simulink model "guidance"  (R2021b)
settings: Solver=VariableStepAuto  StartTime=0.0  StopTime=50  RelTol=1e-3
values from neighbouring files (symbols this model uses):
  A_R = b^2/S    (= 3.125)    [tailsitterParam.m]
  b = [b1;b2;b3;b4;b5;b4;b3]    [tailsitterParam.m]
  c = [c1;c2;c3;c3;c3;c3;c3]    [tailsitterParam.m]
  C_D0 = 0.02    [tailsitterParam.m]
  C_D_R = 1.1    [tailsitterParam.m]
  C_M_coeff = polyfit(C_M_alpha(:,1), C_M_alpha(:,2),3)    [tailsitterParam.m]
  Cl_alpha = (2*pi*cos(Lambda))/(2*cos(Lambda)/A_R + sqrt(1 + (2*cos(Lambda)/A_R)^2))    [tailsitterParam.m]
  d = cat(2,p_d,p_d)    [tailsitterParam.m]
  g = -9.82    [tailsitterParam.m]
  Ic = [Ix 0 -Ixz;0 Iy 0;-Ixz 0 Iz]    [tailsitterParam.m]
  INIT_ETA = [0.5;0;0.5;axang2quat([0 1 0 -1.572])']    [guidanceParams.m]
  Ith = 1.6*10^(-6)    (= 1.6e-06)    [tailsitterParam.m]
  k0 = 0.87    [tailsitterParam.m]
  Kp_o = eye(3)*2    [controllerParams.m]
  Kp_p = eye(3)*5    [controllerParams.m]
  Kv_o = eye(3)*3    [controllerParams.m]
  Kv_p = eye(3)*3    [controllerParams.m]
  l = 0.145    [tailsitterParam.m]
  li = cat(2,lr,ll)    [tailsitterParam.m]
  m = 0.21    [tailsitterParam.m]
  M = [m * eye(3,3) zeros(3,3);zeros(3,3) Ic]    [tailsitterParam.m]
  M_inv = inv(M)    [tailsitterParam.m]
  Omega_max = 1500    [tailsitterParam.m]
  pm = cat(2,prm,plm)    [tailsitterParam.m]
  r_B = r_B./1000    [tailsitterParam.m]
  R_eleb1 = axang2rotm([0 0 1 -0.16349])    [tailsitterParam.m]
  R_eleb2 = axang2rotm([0 0 1 0.15331])    [tailsitterParam.m]
  rho = 1.225    [tailsitterParam.m]
  rp = 0.0625    [tailsitterParam.m]
  rv_B = rv_B./1000    [tailsitterParam.m]
  SLERP_a = flip(SLERP_B \ SLERP_bconstraints)    [guidanceParams.m]
  tf_a = [(1/wn) (1+2*damp) (1+2*damp)*wn wn^2]    [guidanceParams.m]
  tf_b = [wn^2]    [guidanceParams.m]
  wpts = [wpts_p;wpts_qs]    [guidanceParams.m]
libraries: simulink_extras x3, simulink x2, dspswit3 x1, vrlib x1
settings Model: Creator=Thobi  LastModifiedBy=Thobi

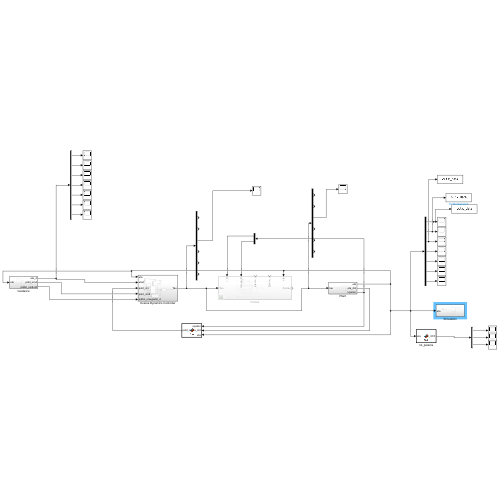
[thumbnail: Simulink's stored preview of the top-level diagram]
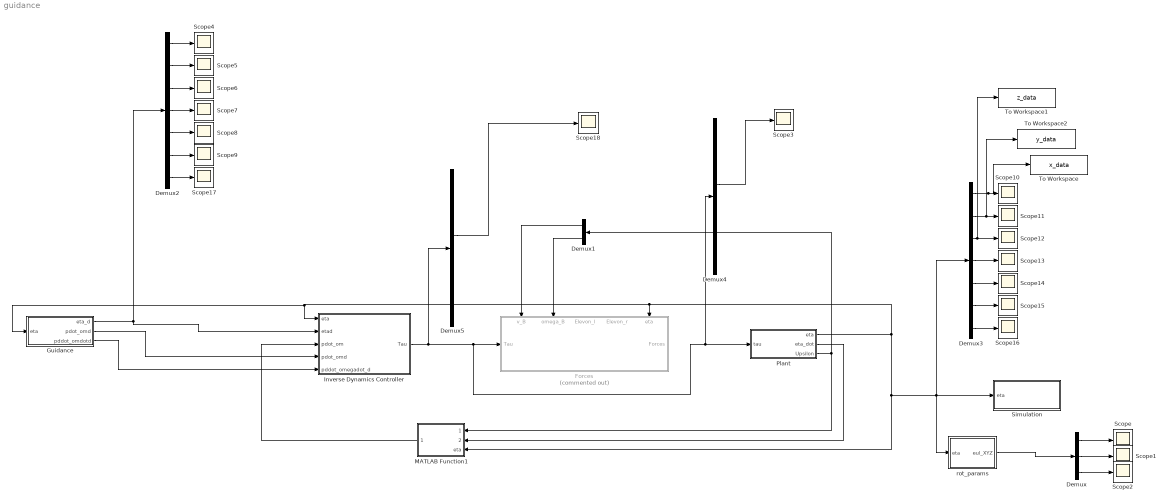
== system guidance ==
  Demux : Demux  Outputs=3
  Demux1 : Demux  Outputs=2
  Demux2 : Demux  Outputs=7
  Demux3 : Demux  Outputs=7
  Demux4 : Demux  Outputs=6
  Demux5 : Demux  Outputs=6
  Forces : Subsystem  Commented=on
      settings: PortSchema="{\"entries\":[{\"content\":{\"sides\":[{\"content\":{\"connectorIds\":[\"In1\"]},\"type\":\"ConnectorPlacement.EquallySpacedRectSide\",\"uuid\":\"b69eaf1b-34d3-48b5-a479-e73058574737\"},{\"content\":{\"connectorIds\":[\"Out1\"],\"side\":\"RIGHT\"},\"type\":\"ConnectorPlacement.EquallySpacedRectSide\",\"uuid\":\"360c4a31-c3bb-45fe-b4f9-363a1910a025\"},{\"content\":{\"connectorIds\":[\"In2\",\"In3\",\"In4\",\"In5\",\"In6\"],\"side\":\"TOP\"},\"type\":\"ConnectorPlacement.EquallySpacedRectSide\",\"uuid\":\"c1210f58-2836-4525-bf47-18b3ef4457c4\"}]},\"type\":\"ConnectorPlacement.EquallySpacedConnector\",\"uuid\":\"84dfde55-8f7b-46f6-8c53-c0c170e7b308\"}],\"packageUris\":[\"http://schema.mathworks.com/mf0/Connector/R2020b\"],\"version\":\"1.0\"}"
  Guidance : Subsystem
  Inverse Dynamics Controller : Subsystem
  MATLAB Function1 : MATLAB Function  TreatAsAtomicUnit=on
  Plant : Subsystem
  Scope{,1..18} (19 alike) : Scope
  Simulation : Subsystem
  To Workspace : ToWorkspace  VariableName=x_data  SaveFormat=Timeseries  SampleTime=-1
  To Workspace1 : ToWorkspace  VariableName=z_data  SaveFormat=Timeseries  SampleTime=-1
  To Workspace2 : ToWorkspace  VariableName=y_data  SaveFormat=Timeseries  SampleTime=-1
  rot_params : MATLAB Function  TreatAsAtomicUnit=on
  wires:
  Plant/2(eta_dot) -> MATLAB Function1/2(eta_dot)
  Plant/3(Upsilon) -> MATLAB Function1/1(upsilon), Demux1/1
  MATLAB Function1/1(pdot_om) -> Inverse Dynamics Controller/3(pdot_om)
  Demux3/1 -> To Workspace/1, Scope10/1
  Demux3/2 -> To Workspace2/1, Scope11/1
  Demux3/3 -> To Workspace1/1, Scope12/1
  Demux3/4 -> Scope13/1
  Demux3/5 -> Scope14/1
  Demux3/6 -> Scope15/1
  Demux3/7 -> Scope16/1
  rot_params/1(eul_XYZ) -> Demux/1
  Demux/1 -> Scope/1
  Demux/2 -> Scope1/1
  Demux/3 -> Scope2/1
  Guidance/2(pdot_omd) -> Inverse Dynamics Controller/4(pdot_omd)
  Plant/1(eta) -> MATLAB Function1/3(eta), rot_params/1(eta), Simulation/1(eta), Demux3/1, Forces/6(eta), Guidance/1(eta), Inverse Dynamics Controller/1(eta)
  Demux2/5 -> Scope8/1
  Demux2/4 -> Scope7/1
  Demux2/3 -> Scope6/1
  Demux2/6 -> Scope9/1
  Demux2/1 -> Scope4/1
  Demux2/2 -> Scope5/1
  Guidance/1(eta_d) -> Inverse Dynamics Controller/2(etad), Demux2/1
  Demux2/7 -> Scope17/1
  Inverse Dynamics Controller/1(Tau) -> Demux5/1, Demux4/1, Plant/1(tau), Forces/1(Tau)
  Demux1/1 -> Forces/2(v_B)
  Demux1/2 -> Forces/3(omega_B)
  Demux5/3 -> Scope18/1
  Guidance/3(pddot_omdotd) -> Inverse Dynamics Controller/5(pddot_omegadot_d)
  Demux4/3 -> Scope3/1

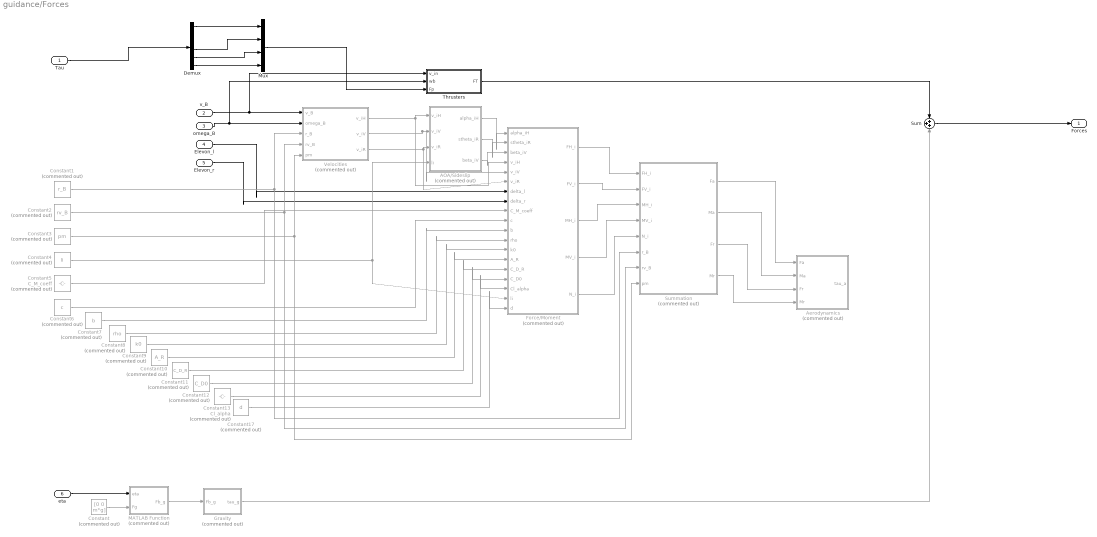
== system guidance/Forces ==
  Tau : Inport
  v_B : Inport  Port=2
  omega_B : Inport  Port=3
  Elevon_l : Inport  Port=4
  Elevon_r : Inport  Port=5
  eta : Inport  Port=6
  AOA/Sideslip : MATLAB Function  Commented=on  TreatAsAtomicUnit=on
  Aerodynamics : MATLAB Function  Commented=on  TreatAsAtomicUnit=on
  Constant : Constant  Commented=on  Value=[0 0 m*g]
  Constant1 : Constant  Commented=on  Value=r_B
  Constant10 : Constant  Commented=on  Value=A_R
  Constant11 : Constant  Commented=on  Value=C_D_R
  Constant12 : Constant  Commented=on  Value=C_D0
  Constant13 : Constant  Commented=on  Value=Cl_alpha
  Constant17 : Constant  Commented=on  Value=d
  Constant2 : Constant  Commented=on  Value=rv_B
  Constant3 : Constant  Commented=on  Value=pm
  Constant4 : Constant  Commented=on  Value=li
  Constant5 : Constant  Commented=on  Value=C_M_coeff
  Constant6 : Constant  Commented=on  Value=c
  Constant7 : Constant  Commented=on  Value=b
  Constant8 : Constant  Commented=on  Value=rho
  Constant9 : Constant  Commented=on  Value=k0
  Demux : Demux  Outputs=6
  Force/Moment : MATLAB Function  Commented=on  TreatAsAtomicUnit=on
  Gravity : MATLAB Function  Commented=on  TreatAsAtomicUnit=on
  MATLAB Function : MATLAB Function  Commented=on  TreatAsAtomicUnit=on
  Mux : Mux
  Sum : Sum  Inputs=+++
  Summation : MATLAB Function  Commented=on  TreatAsAtomicUnit=on
  Thrusters : Subsystem
  Velocities : MATLAB Function  Commented=on  TreatAsAtomicUnit=on
  Forces : Outport
  wires:
  v_B/1 -> Thrusters/1(v_in), Velocities/1(v_B)
  Velocities/1(v_iH) -> AOA/Sideslip/1(v_iH), Force/Moment/4(v_iH)
  Velocities/2(v_iV) -> Force/Moment/5(v_iV), AOA/Sideslip/2(v_iV)
  Velocities/3(v_iR) -> Force/Moment/6(v_iR), AOA/Sideslip/3(v_iR)
  AOA/Sideslip/1(alpha_iH) -> Force/Moment/1(alpha_iH)
  AOA/Sideslip/2(stheta_iR) -> Force/Moment/2(stheta_iR)
  AOA/Sideslip/3(beta_iV) -> Force/Moment/3(beta_iV)
  Force/Moment/1(FH_i) -> Summation/1(FH_i)
  Force/Moment/2(FV_i) -> Summation/2(FV_i)
  Force/Moment/3(MH_i) -> Summation/3(MH_i)
  Force/Moment/4(MV_i) -> Summation/4(MV_i)
  Force/Moment/5(N_i) -> Summation/5(N_i)
  Summation/1(Fa) -> Aerodynamics/1(Fa)
  Summation/2(Ma) -> Aerodynamics/2(Ma)
  Summation/3(Fr) -> Aerodynamics/3(Fr)
  Summation/4(Mr) -> Aerodynamics/4(Mr)
  Sum/1 -> Forces/1
  Elevon_l/1 -> Force/Moment/7(delta_l)
  Elevon_r/1 -> Force/Moment/8(delta_r)
  Constant/1 -> MATLAB Function/2(Fg)
  Constant1/1 -> Summation/6(r_B), Velocities/3(r_B)
  Constant2/1 -> Velocities/4(rv_B), Summation/7(rv_B)
  Constant3/1 -> Velocities/5(pm), Summation/8(pm)
  Constant4/1 -> Force/Moment/18(li), AOA/Sideslip/4(li)
  Constant5/1 -> Force/Moment/9(C_M_coeff)
  Constant6/1 -> Force/Moment/10(c)
  Constant7/1 -> Force/Moment/11(b)
  Constant8/1 -> Force/Moment/12(rho)
  Constant9/1 -> Force/Moment/13(k0)
  Constant10/1 -> Force/Moment/14(A_R)
  Constant11/1 -> Force/Moment/15(C_D_R)
  Constant12/1 -> Force/Moment/16(C_D0)
  Constant13/1 -> Force/Moment/17(Cl_alpha)
  Thrusters/1(FT) -> Sum/1
  Constant17/1 -> Force/Moment/19(d)
  omega_B/1 -> Thrusters/2(wb), Velocities/2(omega_B)
  Tau/1 -> Demux/1
  Demux/1 -> Mux/1
  Demux/4 -> Mux/2
  Demux/5 -> Mux/3
  Demux/6 -> Mux/4
  Mux/1 -> Thrusters/3(Fp)
  eta/1 -> MATLAB Function/1(eta)
  MATLAB Function/1(Fb_g) -> Gravity/1(Fb_g)
  Gravity/1(tau_g) -> Sum/3

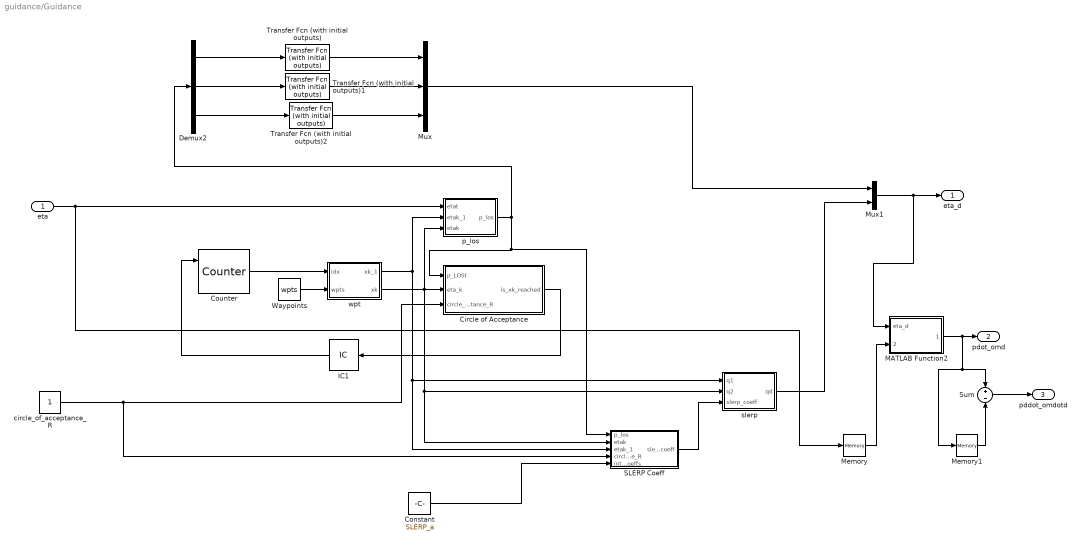
== system guidance/Guidance ==
  eta : Inport
  Circle of Acceptance : MATLAB Function  TreatAsAtomicUnit=on
  Constant : Constant  Value=SLERP_a
  Counter : dspswit3/Counter  Direction=Up  CountEvent=Rising edge  CounterSize=User defined  MaxCount=1000  InitialCount=1  Output=Count  HitValue=32  ResetInput=on  SamplesPerFrame=1  Ts=1  CntDtype=uint32  HitDtype=Logical
  Demux2 : Demux  Outputs=3
  IC1 : InitialCondition  Value=0
  MATLAB Function2 : MATLAB Function  TreatAsAtomicUnit=on
  Memory : Memory  InitialCondition=INIT_ETA
  Memory1 : Memory  InitialCondition=[0;0;0;0;0;0]
  Mux : Mux  Inputs=3
  Mux1 : Mux  Inputs=2
  SLERP Coeff : MATLAB Function  TreatAsAtomicUnit=on
  Sum : Sum  Inputs=+-
  Transfer Fcn (with initial outputs) : simulink_extras/Additional Linear/Transfer Fcn (with initial outputs)  N=tf_b  D=tf_a  Y0=INIT_ETA(1)  U0=INIT_ETA(1)
  Transfer Fcn (with initial outputs)1 : simulink_extras/Additional Linear/Transfer Fcn (with initial outputs)  N=tf_b  D=tf_a  Y0=INIT_ETA(2)  U0=INIT_ETA(2)
  Transfer Fcn (with initial outputs)2 : simulink_extras/Additional Linear/Transfer Fcn (with initial outputs)  N=tf_b  D=tf_a  Y0=INIT_ETA(3)  U0=INIT_ETA(3)
  Waypoints : Constant  Value=wpts
  circle_of_acceptance_R : Constant
  p_los : MATLAB Function  TreatAsAtomicUnit=on
  slerp : MATLAB Function  TreatAsAtomicUnit=on
  wpt : MATLAB Function  TreatAsAtomicUnit=on
  eta_d : Outport
  pdot_omd : Outport  Port=2
  pddot_omdotd : Outport  Port=3
  wires:
  Counter/1 -> wpt/1(idx)
  circle_of_acceptance_R/1 -> SLERP Coeff/4(circle_of_acceptance_R), Circle of Acceptance/3(circle_of_acceptance_R)
  wpt/1(xk_1) -> p_los/2(etak_1), SLERP Coeff/3(etak_1), slerp/1(q1)
  Waypoints/1 -> wpt/2(wpts)
  p_los/1(p_los) -> Demux2/1, SLERP Coeff/1(p_los), Circle of Acceptance/1(p_LOSt)
  Circle of Acceptance/1(is_xk_reached) -> IC1/1
  wpt/2(xk) -> slerp/2(q2), SLERP Coeff/2(etak), p_los/3(etak), Circle of Acceptance/2(eta_k)
  IC1/1 -> Counter/1
  eta/1 -> Memory/1, p_los/1(etat)
  Mux1/1 -> MATLAB Function2/1(eta_d), eta_d/1
  SLERP Coeff/1(slerp_coeff) -> slerp/3(slerp_coeff)
  slerp/1(qd) -> Mux1/2
  Constant/1 -> SLERP Coeff/5(interpolation_coeffs)
  Memory/1 -> MATLAB Function2/2(eta_d_1)
  MATLAB Function2/1(pdot_omd) -> Sum/1, Memory1/1, pdot_omd/1
  Mux/1 -> Mux1/1
  Demux2/1 -> Transfer Fcn (with initial outputs)/1
  Transfer Fcn (with initial outputs)/1 -> Mux/1
  Transfer Fcn (with initial outputs)1/1 -> Mux/2
  Demux2/2 -> Transfer Fcn (with initial outputs)1/1
  Demux2/3 -> Transfer Fcn (with initial outputs)2/1
  Transfer Fcn (with initial outputs)2/1 -> Mux/3
  Sum/1 -> pddot_omdotd/1
  Memory1/1 -> Sum/2

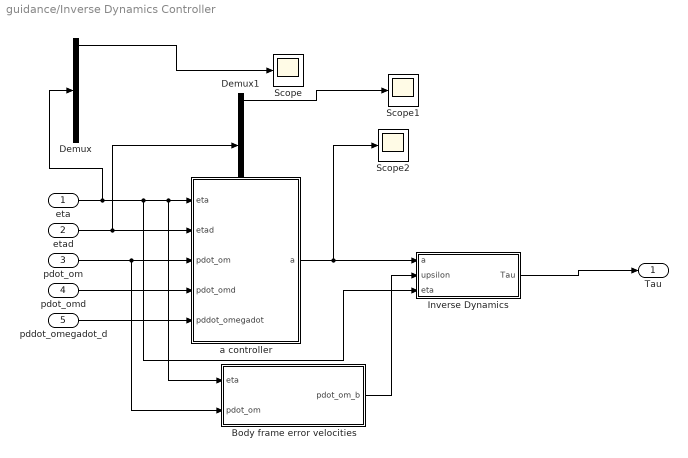
== system guidance/Inverse Dynamics Controller ==
  eta : Inport
  etad : Inport  Port=2
  pdot_om : Inport  Port=3
  pdot_omd : Inport  Port=4
  pddot_omegadot_d : Inport  Port=5
  Body frame error velocities : MATLAB Function  TreatAsAtomicUnit=on
  Demux : Demux  Outputs=7
  Demux1 : Demux  Outputs=7
  Inverse Dynamics : Subsystem
  Scope : Scope
  Scope1 : Scope
  Scope2 : Scope
  a controller : Subsystem
  Tau : Outport
  wires:
  a controller/1(a) -> Scope2/1, Inverse Dynamics/1(a)
  Inverse Dynamics/1(Tau) -> Tau/1
  pddot_omegadot_d/1 -> a controller/5(pddot_omegadot)
  pdot_omd/1 -> a controller/4(pdot_omd)
  pdot_om/1 -> Body frame error velocities/2(pdot_om), a controller/3(pdot_om)
  etad/1 -> Demux1/1, a controller/2(etad)
  eta/1 -> Demux/1, Inverse Dynamics/3(eta), Body frame error velocities/1(eta), a controller/1(eta)
  Body frame error velocities/1(pdot_om_b) -> Inverse Dynamics/2(upsilon)
  Demux/1 -> Scope/1
  Demux1/1 -> Scope1/1

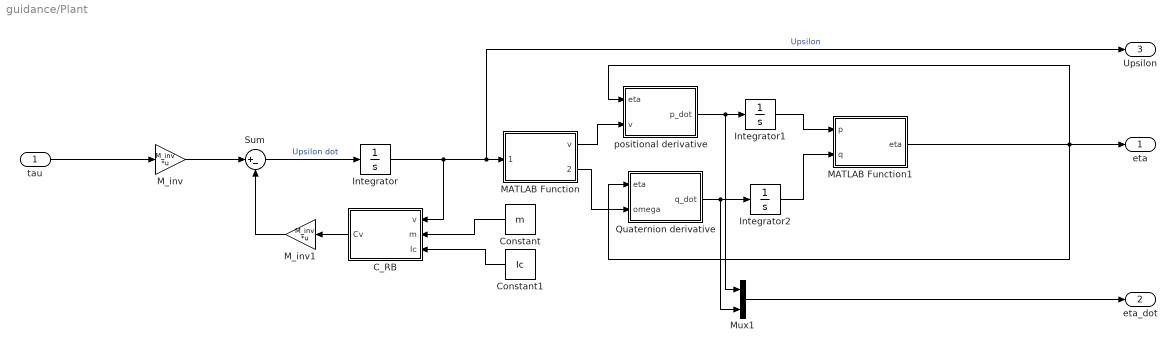
== system guidance/Plant ==
  tau : Inport
  C_RB : MATLAB Function  TreatAsAtomicUnit=on
  Constant : Constant  Value=m
  Constant1 : Constant  Value=Ic
  Integrator : Integrator  InitialCondition=[0;0;0;0;0;0]
  Integrator1 : Integrator  InitialCondition=INIT_ETA(1:3)
  Integrator2 : Integrator  InitialCondition=INIT_ETA(4:7)
  MATLAB Function : MATLAB Function  TreatAsAtomicUnit=on
  MATLAB Function1 : MATLAB Function  TreatAsAtomicUnit=on
  M_inv : Gain  Gain=M_inv  Multiplication=Matrix(K*u) (u vector)
  M_inv1 : Gain  Gain=M_inv  Multiplication=Matrix(K*u) (u vector)
  Mux1 : Mux  Inputs=2
  Quaternion derivative : MATLAB Function  TreatAsAtomicUnit=on
  Sum : Sum  Inputs=|+-
  positional derivative : MATLAB Function  TreatAsAtomicUnit=on
  eta : Outport
  eta_dot : Outport  Port=2
  Upsilon : Outport  Port=3
  wires:
  M_inv/1 -> Sum/1
  Constant/1 -> C_RB/2(m)
  M_inv1/1 -> Sum/2
  tau/1 -> M_inv/1
  Integrator/1 -> C_RB/1(v), MATLAB Function/1(upsilon), Upsilon/1  "Upsilon"
  Constant1/1 -> C_RB/3(Ic)
  C_RB/1(Cv) -> M_inv1/1
  Sum/1 -> Integrator/1  "Upsilon dot"
  positional derivative/1(p_dot) -> Mux1/1, Integrator1/1
  Integrator1/1 -> MATLAB Function1/1(p)
  Quaternion derivative/1(q_dot) -> Mux1/2, Integrator2/1
  Integrator2/1 -> MATLAB Function1/2(q)
  Mux1/1 -> eta_dot/1
  MATLAB Function/1(v) -> positional derivative/2(v)
  MATLAB Function/2(omega) -> Quaternion derivative/2(omega)
  MATLAB Function1/1(eta) -> positional derivative/1(eta), eta/1, Quaternion derivative/1(eta)

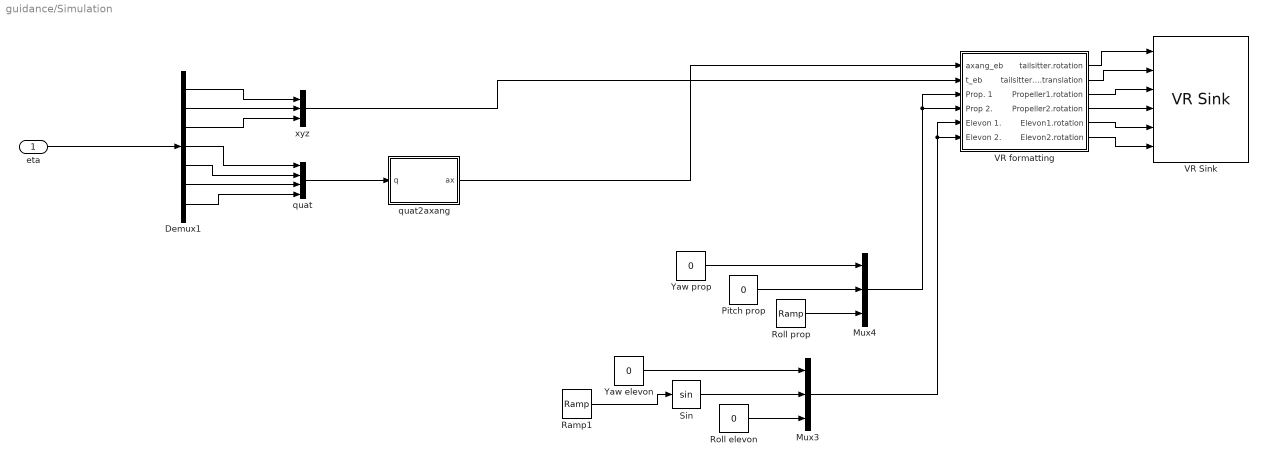
== system guidance/Simulation ==
  eta : Inport
  Demux1 : Demux  Outputs=7
  Mux3 : Mux  Inputs=3
  Mux4 : Mux  Inputs=3
  Pitch prop : Constant  Value=0
  Ramp1 : simulink/Sources/Ramp  slope=1  start=0  InitialOutput=0
  Roll elevon : Constant  Value=0
  Roll prop : simulink/Sources/Ramp  slope=1  start=0  InitialOutput=0
  Sin : Trigonometry
  VR Sink : vrlib/VR Sink  InstantiateOnLoad=on  SampleTime=0.1  ViewEnable=on  RemoteChange=off  RemoteView=on  FieldsWritten=UAV.rotation.4.1.1.double#UAV.translation.3.1.1.double#Propeller1.rotation.4.1.1.double#Propeller2.rotation.4.1.1.double#Elevon1.rotation.4.1.1.double#Elevon2.rotation.4.1.1.double  WorldFileName=tailsitter_VR_simple.x3d  AutoView=off  VideoDimensions=[]  AllowVariableSize=off
  VR formatting : Subsystem
  Yaw elevon : Constant  Value=0
  Yaw prop : Constant  Value=0
  quat : Mux
  quat2axang : MATLAB Function  TreatAsAtomicUnit=on
  xyz : Mux  Inputs=3
  wires:
  eta/1 -> Demux1/1
  quat/1 -> quat2axang/1(q)
  quat2axang/1(ax) -> VR formatting/1(axang_eb)
  Demux1/7 -> quat/4
  Mux3/1 -> VR formatting/6(Elevon 2.), VR formatting/5(Elevon 1.)
  Mux4/1 -> VR formatting/4(Prop 2.), VR formatting/3("Prop. 1 ")
  VR formatting/6(Elevon2.rotation) -> VR Sink/6
  Demux1/3 -> xyz/3
  Demux1/1 -> xyz/1
  VR formatting/3(Propeller1.rotation) -> VR Sink/3
  Yaw elevon/1 -> Mux3/1
  Roll elevon/1 -> Mux3/3
  VR formatting/4(Propeller2.rotation) -> VR Sink/4
  Roll prop/1 -> Mux4/3
  Yaw prop/1 -> Mux4/1
  Demux1/6 -> quat/3
  Demux1/5 -> quat/2
  VR formatting/1(tailsitter.rotation) -> VR Sink/1
  Sin/1 -> Mux3/2
  Demux1/4 -> quat/1
  VR formatting/5(Elevon1.rotation) -> VR Sink/5
  Pitch prop/1 -> Mux4/2
  Ramp1/1 -> Sin/1
  Demux1/2 -> xyz/2
  xyz/1 -> VR formatting/2(t_eb)
  VR formatting/2(tailsitter.translation) -> VR Sink/2

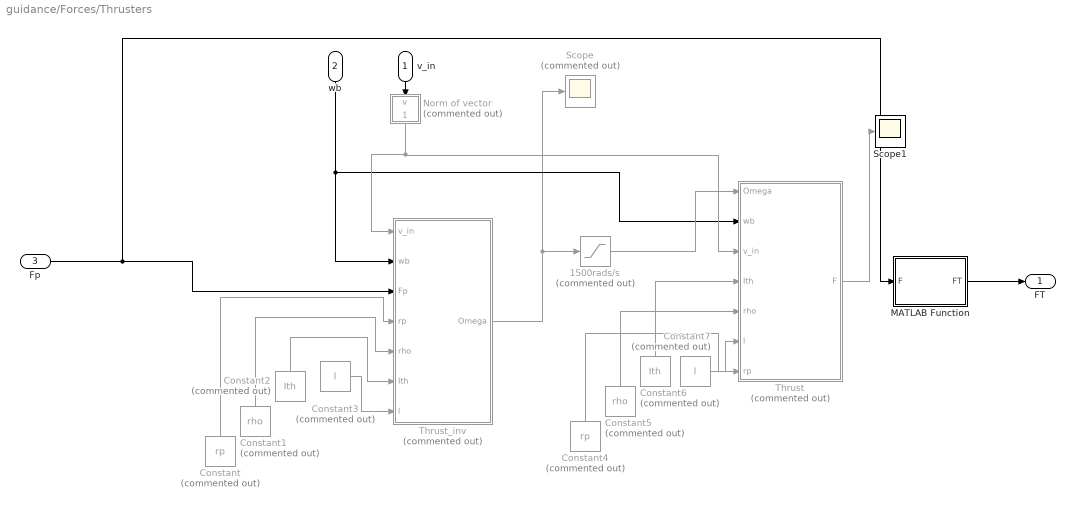
== system guidance/Forces/Thrusters ==
  v_in : Inport
  wb : Inport  Port=2
  Fp : Inport  Port=3  PortDimensions=4
  1500rads/s : Saturate  Commented=on  UpperLimit=Omega_max  LowerLimit=-Omega_max
  Constant : Constant  Commented=on  Value=rp
  Constant1 : Constant  Commented=on  Value=rho
  Constant2 : Constant  Commented=on  Value=Ith
  Constant3 : Constant  Commented=on  Value=l
  Constant4 : Constant  Commented=on  Value=rp
  Constant5 : Constant  Commented=on  Value=rho
  Constant6 : Constant  Commented=on  Value=Ith
  Constant7 : Constant  Commented=on  Value=l
  MATLAB Function : MATLAB Function  TreatAsAtomicUnit=on
  Norm of vector : MATLAB Function  Commented=on  TreatAsAtomicUnit=on
  Scope : Scope  Commented=on
  Scope1 : Scope
  Thrust : MATLAB Function  Commented=on  TreatAsAtomicUnit=on
  Thrust_inv : MATLAB Function  Commented=on  TreatAsAtomicUnit=on
  FT : Outport
  wires:
  Thrust/1(F) -> Scope1/1
  Thrust_inv/1(Omega) -> Scope/1, 1500rads/s/1
  wb/1 -> Thrust_inv/2(wb), Thrust/2(wb)
  Constant4/1 -> Thrust/7(rp)
  Constant5/1 -> Thrust/5(rho)
  Constant6/1 -> Thrust/4(Ith)
  Constant7/1 -> Thrust/6(l)
  MATLAB Function/1(FT) -> FT/1
  v_in/1 -> Norm of vector/1(v)
  Norm of vector/1(v_norm) -> Thrust_inv/1(v_in), Thrust/3(v_in)
  1500rads/s/1 -> Thrust/1(Omega)
  Constant3/1 -> Thrust_inv/7(l)
  Constant/1 -> Thrust_inv/4(rp)
  Constant2/1 -> Thrust_inv/6(Ith)
  Constant1/1 -> Thrust_inv/5(rho)
  Fp/1 -> MATLAB Function/1(F), Thrust_inv/3(Fp)

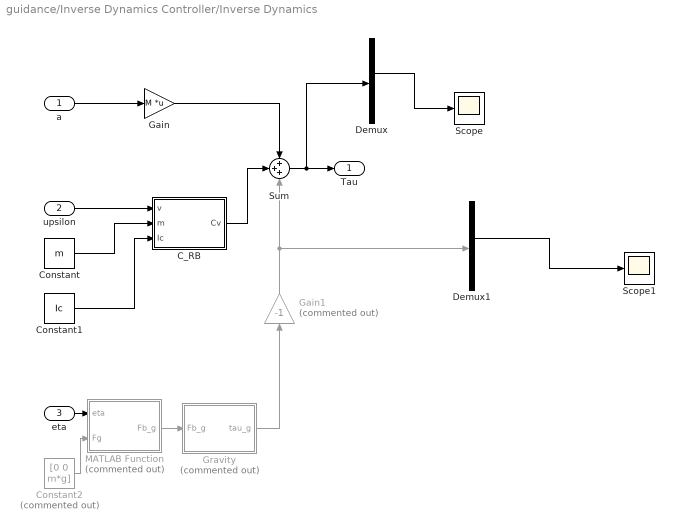
== system guidance/Inverse Dynamics Controller/Inverse Dynamics ==
  a : Inport
  upsilon : Inport  Port=2
  eta : Inport  Port=3
  C_RB : MATLAB Function  TreatAsAtomicUnit=on
  Constant : Constant  Value=m
  Constant1 : Constant  Value=Ic
  Constant2 : Constant  Commented=on  Value=[0 0 m*g]
  Demux : Demux  Outputs=6
  Demux1 : Demux  Outputs=6
  Gain : Gain  Gain=M  Multiplication=Matrix(K*u) (u vector)
  Gain1 : Gain  Commented=on  Gain=-1
  Gravity : MATLAB Function  Commented=on  TreatAsAtomicUnit=on
  MATLAB Function : MATLAB Function  Commented=on  TreatAsAtomicUnit=on
  Scope : Scope
  Scope1 : Scope
  Sum : Sum  Inputs=+++
  Tau : Outport
  wires:
  a/1 -> Gain/1
  upsilon/1 -> C_RB/1(v)
  Constant/1 -> C_RB/2(m)
  Constant1/1 -> C_RB/3(Ic)
  Gain/1 -> Sum/1
  C_RB/1(Cv) -> Sum/2
  Sum/1 -> Demux/1, Tau/1
  Demux/3 -> Scope/1
  eta/1 -> MATLAB Function/1(eta)
  MATLAB Function/1(Fb_g) -> Gravity/1(Fb_g)
  Constant2/1 -> MATLAB Function/2(Fg)
  Gravity/1(tau_g) -> Gain1/1
  Gain1/1 -> Sum/3, Demux1/1
  Demux1/3 -> Scope1/1

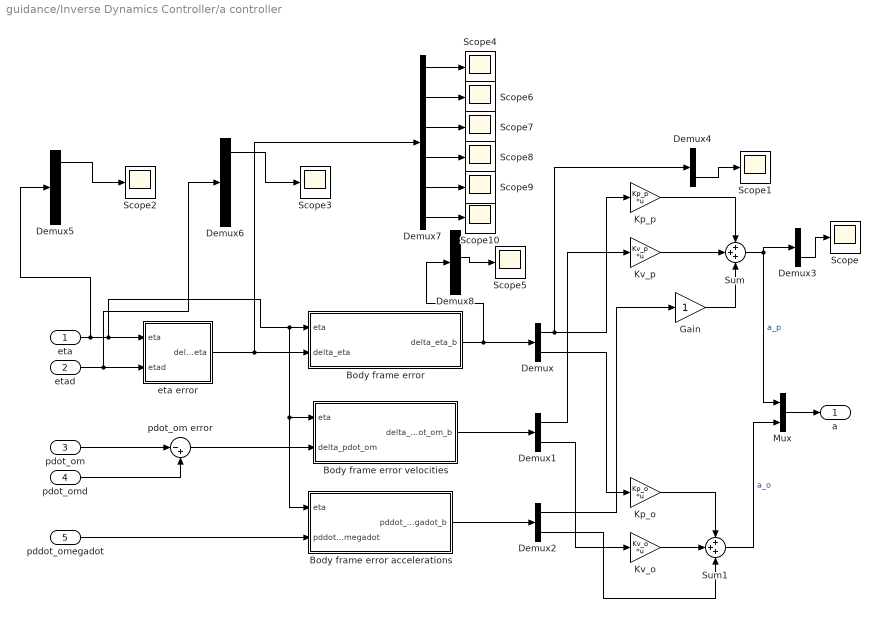
== system guidance/Inverse Dynamics Controller/a controller ==
  eta : Inport
  etad : Inport  Port=2
  pdot_om : Inport  Port=3
  pdot_omd : Inport  Port=4
  pddot_omegadot : Inport  Port=5
  Body frame error : MATLAB Function  TreatAsAtomicUnit=on
  Body frame error accelerations : MATLAB Function  TreatAsAtomicUnit=on
  Body frame error velocities : MATLAB Function  TreatAsAtomicUnit=on
  Demux : Demux  Outputs=2
  Demux1 : Demux  Outputs=2
  Demux2 : Demux  Outputs=2
  Demux3 : Demux  Outputs=3
  Demux4 : Demux  Outputs=3
  Demux5 : Demux  Outputs=6
  Demux6 : Demux  Outputs=7
  Demux7 : Demux  Outputs=6
  Demux8 : Demux  Outputs=6
  Gain : Gain
  Kp_o : Gain  Gain=Kp_o  Multiplication=Matrix(K*u) (u vector)
  Kp_p : Gain  Gain=Kp_p  Multiplication=Matrix(K*u) (u vector)
  Kv_o : Gain  Gain=Kv_o  Multiplication=Matrix(K*u) (u vector)
  Kv_p : Gain  Gain=Kv_p  Multiplication=Matrix(K*u) (u vector)
  Mux : Mux  Inputs=2
  Scope{,1..10} (11 alike) : Scope
  Sum : Sum  Inputs=+++
  Sum1 : Sum  Inputs=+++
  eta error : MATLAB Function  TreatAsAtomicUnit=on
  pdot_om error : Sum  Inputs=|-+
  a : Outport
  wires:
  etad/1 -> Demux6/1, eta error/2(etad)
  eta/1 -> Demux5/1, Body frame error accelerations/1(eta), Body frame error velocities/1(eta), Body frame error/1(eta), eta error/1(eta)
  pdot_omd/1 -> pdot_om error/2
  pdot_om/1 -> pdot_om error/1
  Demux/1 -> Demux4/1, Kp_p/1
  Demux1/1 -> Kv_p/1
  Kp_p/1 -> Sum/1
  Kv_p/1 -> Sum/2
  Demux2/1 -> Gain/1
  Mux/1 -> a/1
  Sum/1 -> Mux/1, Demux3/1  "a_p"
  Demux/2 -> Kp_o/1
  Demux1/2 -> Kv_o/1
  Demux2/2 -> Sum1/3
  Kp_o/1 -> Sum1/1
  Kv_o/1 -> Sum1/2
  Sum1/1 -> Mux/2  "a_o"
  eta error/1(delta_eta) -> Demux7/1, Body frame error/2(delta_eta)
  Body frame error/1(delta_eta_b) -> Demux8/1, Demux/1
  pdot_om error/1 -> Body frame error velocities/2(delta_pdot_om)
  Body frame error velocities/1(delta_pdot_om_b) -> Demux1/1
  pddot_omegadot/1 -> Body frame error accelerations/2(pddot_omegadot)
  Body frame error accelerations/1(pddot_omegadot_b) -> Demux2/1
  Gain/1 -> Sum/3
  Demux3/3 -> Scope/1
  Demux4/3 -> Scope1/1
  Demux5/1 -> Scope2/1
  Demux6/1 -> Scope3/1
  Demux7/1 -> Scope4/1
  Demux8/3 -> Scope5/1
  Demux7/2 -> Scope6/1
  Demux7/3 -> Scope7/1
  Demux7/4 -> Scope8/1
  Demux7/5 -> Scope9/1
  Demux7/6 -> Scope10/1

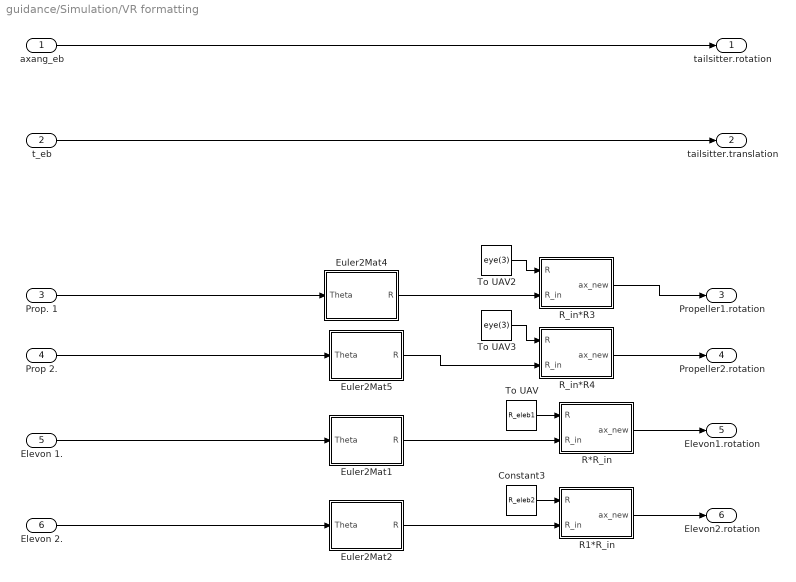
== system guidance/Simulation/VR formatting ==
  axang_eb : Inport
  t_eb : Inport  Port=2
  "Prop. 1 " : Inport  Port=3
  Prop 2. : Inport  Port=4
  Elevon 1. : Inport  Port=5
  Elevon 2. : Inport  Port=6
  Constant3 : Constant  Value=R_eleb2
  Euler2Mat1 : MATLAB Function  TreatAsAtomicUnit=on
  Euler2Mat2 : MATLAB Function  TreatAsAtomicUnit=on
  Euler2Mat4 : MATLAB Function  TreatAsAtomicUnit=on
  Euler2Mat5 : MATLAB Function  TreatAsAtomicUnit=on
  R*R_in : MATLAB Function  TreatAsAtomicUnit=on
  R1*R_in : MATLAB Function  TreatAsAtomicUnit=on
  R_in*R3 : MATLAB Function  TreatAsAtomicUnit=on
  R_in*R4 : MATLAB Function  TreatAsAtomicUnit=on
  To UAV : Constant  Value=R_eleb1
  To UAV2 : Constant  Value=eye(3)
  To UAV3 : Constant  Value=eye(3)
  tailsitter.rotation : Outport
  tailsitter.translation : Outport  Port=2
  Propeller1.rotation : Outport  Port=3
  Propeller2.rotation : Outport  Port=4
  Elevon1.rotation : Outport  Port=5
  Elevon2.rotation : Outport  Port=6
  wires:
  t_eb/1 -> tailsitter.translation/1
  "Prop. 1 "/1 -> Euler2Mat4/1(Theta)
  Elevon 1./1 -> Euler2Mat1/1(Theta)
  Elevon 2./1 -> Euler2Mat2/1(Theta)
  Euler2Mat1/1(R) -> R*R_in/2(R_in)
  To UAV/1 -> R*R_in/1(R)
  R*R_in/1(ax_new) -> Elevon1.rotation/1
  Euler2Mat2/1(R) -> R1*R_in/2(R_in)
  R1*R_in/1(ax_new) -> Elevon2.rotation/1
  Constant3/1 -> R1*R_in/1(R)
  axang_eb/1 -> tailsitter.rotation/1
  To UAV2/1 -> R_in*R3/1(R)
  Euler2Mat4/1(R) -> R_in*R3/2(R_in)
  R_in*R3/1(ax_new) -> Propeller1.rotation/1
  Prop 2./1 -> Euler2Mat5/1(Theta)
  R_in*R4/1(ax_new) -> Propeller2.rotation/1
  To UAV3/1 -> R_in*R4/1(R)
  Euler2Mat5/1(R) -> R_in*R4/2(R_in)

== matlab function guidance/Inverse Dynamics Controller/a controller/Body frame error ==
  data: eta input; delta_eta input; delta_eta_b output size=6
function delta_eta_b = fcn(eta, delta_eta)
   R = quat2rotm(eta(4:7)');
   delta_eta_b = [R'*delta_eta(1:3); R'*delta_eta(4:6)];
end

== matlab function guidance/Inverse Dynamics Controller/a controller/Body frame error velocities ==
  data: eta input; delta_pdot_om input; delta_pdot_om_b output size=6
function delta_pdot_om_b = fcn(eta, delta_pdot_om)
   R = quat2rotm(eta(4:7)');
   delta_pdot_om_b = [R'*delta_pdot_om(1:3); R'*delta_pdot_om(4:6)];
end

== matlab function guidance/Inverse Dynamics Controller/Inverse Dynamics/C_RB ==
  data: v input; m input; Ic input; Cv output
function Cv = fcn(v, m, Ic)
    w = v(4:6,1);
    w_cross = [0 -w(3) w(2);w(3) 0 -w(1);-w(2) w(1) 0];
    Ic_w = Ic*w;    
    Ic_w_cross = [0 -Ic_w(3) Ic_w(2);Ic_w(3) 0 -Ic_w(1);-Ic_w(2) Ic_w(1) 0];
    C = [m*w_cross zeros(3,3);zeros(3,3) -Ic_w_cross];
    Cv = C*v;
end

== matlab function guidance/Plant/C_RB ==
  data: v input; m input; Ic input; Cv output
function Cv = fcn(v, m, Ic)
    w = v(4:6,1);
    w_cross = [0 -w(3) w(2);w(3) 0 -w(1);-w(2) w(1) 0];
    Ic_w = Ic*w;    
    Ic_w_cross = [0 -Ic_w(3) Ic_w(2);Ic_w(3) 0 -Ic_w(1);-Ic_w(2) Ic_w(1) 0];
    C = [m*w_cross zeros(3,3);zeros(3,3) -Ic_w_cross];
    Cv = C*v;
end

== matlab function guidance/Plant/positional derivative ==
  data: eta input; p_dot output size=3; v input
function p_dot = fcn(eta, v)
    R = quat2rotm(eta(4:7)');
    p_dot = R * v;
end

== matlab function guidance/Plant/Quaternion derivative ==
  data: eta input; q_dot output size=4; omega input
function q_dot = fcn(eta, omega)
    q = quaternion(eta(4:7)');
    q_omega = quaternion([0 omega']);
    
    q_dot_temp = 0.5 * q * q_omega;
    [n, e1, e2, e3] = parts(q_dot_temp);

    q_dot = [n; e1; e2; e3];
end

== matlab function guidance/Inverse Dynamics Controller/a controller/Body frame error accelerations ==
  data: eta input; pddot_omegadot input; pddot_omegadot_b output size=6
function pddot_omegadot_b = fcn(eta, pddot_omegadot)
   R = quat2rotm(eta(4:7)');
   pddot_omegadot_b = [R'*pddot_omegadot(1:3); R'*pddot_omegadot(4:6)];
end

== matlab function guidance/MATLAB Function1 ==
  data: upsilon input; eta_dot input; pdot_om output size=6; eta input
function pdot_om = fcn(upsilon, eta_dot, eta)
    R = quat2rotm(eta(4:7)');
    omega_b = upsilon(4:6);
    
    omega_e = R * omega_b;

    pdot_om = [eta_dot(1:3);omega_e];
end

== matlab function guidance/Plant/MATLAB Function ==
  data: upsilon input; v output; omega output
function [v,omega] = fcn(upsilon)
    v = upsilon(1:3);
    omega = upsilon(4:6);
end

== matlab function guidance/Plant/MATLAB Function1 ==
  data: p input; eta output; q input
function eta = fcn(p, q)
    eta = [p;q];
end

== matlab function guidance/Simulation/VR formatting/Euler2Mat1 ==
  data: Theta input; R output
function R = fcn(Theta)
R = eul2rotm(Theta', "ZYX"); %YAW - PITCH - ROLL
end

== matlab function guidance/Simulation/VR formatting/Euler2Mat2 ==
  data: Theta input; R output
function R = fcn(Theta)
R = eul2rotm(Theta', "ZYX"); %YAW - PITCH - ROLL
end

== matlab function guidance/Forces/AOA//Sideslip ==
  data: v_iH input; alpha_iH output; v_iV input; v_iR input; stheta_iR output; beta_iV output; li input
function [alpha_iH, stheta_iR, beta_iV] = fcn(v_iH, v_iV, v_iR, li)

    alpha_iH = zeros(size(v_iH,2),1);
    for i = 1:size(v_iH,2)
        alpha_iH(i) = atan2(v_iH(3,i),v_iH(1,i));
    end
    
    beta_iV = zeros(size(v_iV,2),1);
    for i = 1:size(v_iV,2)
        beta_iV(i) = atan2(v_iV(2,i),v_iV(1,i));
    end
    
    stheta_iR = zeros(size(v_iR,2),1);
    if norm(v_iR) == 0
        stheta_iR = zeros(size(v_iR,2),1);
    else
        for i = 1:size(v_iR,2)
            stheta_iR(i) = (norm(cross(v_iR(:,i),li(:,i))))/(norm(v_iR(:,i))*norm(li(:,i)));
        end
    end
end

== matlab function guidance/Simulation/VR formatting/Euler2Mat4 ==
  data: Theta input; R output
function R = fcn(Theta)
R = eul2rotm(Theta', "ZYX"); %YAW - PITCH - ROLL
end

== matlab function guidance/Simulation/VR formatting/Euler2Mat5 ==
  data: Theta input; R output
function R = fcn(Theta)
R = eul2rotm(Theta', "ZYX"); %YAW - PITCH - ROLL
end

== matlab function guidance/Forces/Aerodynamics ==
  data: Fa input size=3; tau_a output size=6; Ma input size=3; Fr input size=3; Mr input size=3
function tau_a = fcn(Fa, Ma, Fr, Mr)

    tau_a = zeros(6,1);
    tau_a(1:3) = Fa + Fr;
    tau_a(4:6) = Ma + Mr;

end

== matlab function guidance/Simulation/VR formatting/R*R_in ==
  data: R input; ax_new output; R_in input
function ax_new = fcn(R, R_in)
    ax_new = rotm2axang(R*R_in)';
end

== matlab function guidance/Simulation/VR formatting/R1*R_in ==
  data: R input; ax_new output; R_in input
function ax_new = fcn(R, R_in)
    ax_new = rotm2axang(R*R_in)';
end

== matlab function guidance/Forces/Force//Moment ==
  data: alpha_iH input; stheta_iR input; beta_iV input; FH_i output; v_iH input; v_iV input; FV_i output; MH_i output; MV_i output; N_i output; v_iR input; delta_l input; delta_r input; C_M_coeff input; c input; b input; rho input; k0 input; A_R input; C_D_R input; C_D0 input; Cl_alpha input; li input; d input
function [FH_i, FV_i, MH_i, MV_i, N_i] = fcn(alpha_iH, stheta_iR, beta_iV, v_iH, v_iV, v_iR, delta_l, delta_r, C_M_coeff, c, b, rho, k0, A_R, C_D_R, C_D0, Cl_alpha, li, d)
    CL = 0;
    FH_i = zeros(3,size(alpha_iH,1));
    MH_i = zeros(3,size(alpha_iH,1));
    for i = 1:size(alpha_iH,1)
        if i == 4
            CL = Cl_alpha*(alpha_iH(1)+delta_l);
        elseif i == 6
            CL = Cl_alpha*(alpha_iH(1)+delta_r);
        else
            CL = Cl_alpha*alpha_iH(1);
        end
        CD = C_D0 + (CL^2)/(pi*k0*A_R);
        FHba_i = [CL*sin(alpha_iH(i))-CD*cos(alpha_iH(i)); 0; -CL*cos(alpha_iH(i))-CD*sin(alpha_iH(i))];
        FH_i(:,i) = (1/2)*rho*b(i)*c(i)*(v_iH(1,i)^2+v_iH(3,i)^2)*FHba_i;
        
        MH_i(:,i) = (1/2)*rho*b(i)*c(i)^2*(v_iH(1,i)^2+v_iH(3,i)^2)*(sum(C_M_coeff*alpha_iH(i)));
    end
    
    CL = 0;
    FV_i = zeros(3,size(beta_iV,1));
    MV_i = zeros(3,size(beta_iV,1));
    for i = 1:size(beta_iV,1)
        CL = Cl_alpha*alpha_iH(1);
        CD = C_D0 + (CL^2)/(pi*k0*A_R);
        FVba_i = [CL*sin(beta_iV(i))-CD*cos(beta_iV(i)); -CL*cos(beta_iV(i))-CD*sin(beta_iV(i)); 0];
        FV_i(:,i) = (1/2)*rho*b(i)*c(i)*(v_iV(1,i)^2+v_iV(2,i))*FVba_i;
        
        MV_i(:,i) = (1/2)*rho*b(i)*c(i)^2*(v_iV(1,i)^2+v_iV(2,i)^2)*(sum(C_M_coeff*alpha_iH(1)));
    end

    N_i = zeros(3,size(stheta_iR,1));
    for i = 1:size(stheta_iR,1)
        N_i(:,i)=(1/2)*rho*v_iR(:,i).^2*li(i)*d(i)*C_D_R*stheta_iR(i)^2;
    end
    
    
end

== matlab function guidance/Simulation/VR formatting/R_in*R3 ==
  data: R input; ax_new output; R_in input
function ax_new = fcn(R, R_in)
    ax_new = rotm2axang(R_in*R)';
end

== matlab function guidance/Guidance/p_los ==
  data: etat input size=7; p_los output size=3; etak_1 input size=7; etak input size=7
function p_los = fcn(etat, etak_1, etak)
    xk = etak(1:3);
    xk_1 = etak_1(1:3);
    xt = etat(1:3);

    p = xk - xk_1;
    pt = xt - xk_1;
    d = (dot(pt,p)/dot(p,p)) * p;
    delta = 0.9;
    v_los = d + delta * p/norm(p);
    if norm(p) < norm(v_los)
        p_los = p + xk_1;
    else
        p_los = v_los + xk_1;
    end
end

== matlab function guidance/Simulation/VR formatting/R_in*R4 ==
  data: R input; ax_new output; R_in input
function ax_new = fcn(R, R_in)
    ax_new = rotm2axang(R_in*R)';
end

== matlab function guidance/Simulation/quat2axang ==
  data: q input; ax output
function ax = fcn(q)
   ax = quat2axang(q');
end

== matlab function guidance/Forces/Gravity ==
  data: Fb_g input; tau_g output
function tau_g = fcn(Fb_g)

    tau_g = zeros(6,1);
    tau_g(1:3,1) = Fb_g;
    

end

== matlab function guidance/Forces/Summation ==
  data: FH_i input; Fa output; FV_i input; MH_i input; MV_i input; N_i input; Ma output; Fr output; Mr output; r_B input; rv_B input; pm input
function [Fa, Ma, Fr, Mr] = fcn(FH_i, FV_i, MH_i, MV_i, N_i, r_B, rv_B, pm)

    Fa = zeros(3,1);
    
    for i = 1:size(FH_i,2)
        Fa = Fa + FH_i(:,i);
    end
    
    for i = 1:size(FV_i,2)
        Fa = Fa + FV_i(:,i);
    end
    
    Ma = zeros(3,1);
    
    for i = 1:size(MH_i,2)
        Ma = Ma + (MH_i(:,i) + cross(r_B(:,i),FH_i(:,i)));
    end
    
    for i = 1:size(MV_i,2)
        Ma = Ma + (MV_i(:,i) + cross(rv_B(:,i),FV_i(:,i)));
    end
    
    Fr = zeros(3,1);
    Mr = zeros(3,1);
    
    for i = 1:size(N_i,2)
        Fr = Fr + N_i(:,i);
        Mr = Mr + cross(pm(:,i),N_i(:,i));
    end


end

== matlab function guidance/Forces/Thrusters/MATLAB Function ==
  data: F input size=4; FT output size=6
function FT = fcn(F)

    FT = zeros(6,1);
    FT(1) = F(1);
    FT(4:6) = F(2:4);
end

== matlab function guidance/Forces/Thrusters/Norm of vector ==
  data: v input; v_norm output
function v_norm = fcn(v)
    v_norm = norm(v);
end

== matlab function guidance/Forces/Thrusters/Thrust ==
  data: Omega input; wb input; v_in input; Ith input; rho input; l input; F output size=4; rp input
function F = fcn(Omega, wb, v_in, Ith, rho, l,  rp)
    %Omega(1) = Omega_Left, Omega(2) = Omega_Right
    F = Thrust_param(Omega, wb, v_in, Ith, l, rho, rp);
end

== matlab function guidance/Forces/Thrusters/Thrust_inv ==
  data: v_in input; wb input; Fp input; rp input; rho input; Ith input; l input; Omega output size=2
function Omega = fcn(v_in, wb, Fp, rp, rho, Ith, l)
    lb = [-1500; 1500];
    ub = [1500; 1500];
    Omega_init = (lb + ub)/2;
    coder. extrinsic('Thrust_inv');
    Omega = zeros(2,1);
    Omega = Thrust_inv(v_in, wb, Fp, rp, rho, Ith, l, Omega_init, lb, ub);
end

== matlab function guidance/Forces/Velocities ==
  data: v_B input; v_iH output; omega_B input; v_iV output; v_iR output; r_B input; rv_B input; pm input
function [v_iH, v_iV, v_iR] = fcn(v_B,omega_B, r_B, rv_B, pm)
    v_w = 0;
    v_iH = zeros(3, size(r_B,2));
    for i = 1:size(r_B,2)
        v_iH(:,i) = v_B + cross(omega_B,r_B(:,i)) + v_w;
    end
    
    v_iV = zeros(3, size(rv_B,2));
    for i = 1:size(rv_B,2)
        v_iV(:,i) = v_B + cross(omega_B,rv_B(:,i)) + v_w;
    end
    
    v_iR = zeros(3, size(pm,2));
    for i = 1:size(pm,2)
        v_iR(:,i) = v_B + cross(omega_B,pm(:,i)) + v_w;
    end
    

end

== matlab function guidance/Guidance/Circle of Acceptance ==
  data: p_LOSt input size=3; is_xk_reached output; eta_k input size=7; circle_of_acceptance_R input
function is_xk_reached = fcn(p_LOSt, eta_k, circle_of_acceptance_R)
    d = norm(eta_k(1:3)-p_LOSt);
   
    is_xk_reached = 0;
    if d <= circle_of_acceptance_R(1)
        is_xk_reached = 1;
    end
end

== matlab function guidance/Forces/MATLAB Function ==
  data: eta input; Fb_g output; Fg input
function Fb_g = fcn(eta, Fg)
    R = quat2rotm(eta(4:7)');
    Fb_g = R' * Fg;
end

== matlab function guidance/Inverse Dynamics Controller/Inverse Dynamics/Gravity ==
  data: Fb_g input; tau_g output
function tau_g = fcn(Fb_g)

    tau_g = zeros(6,1);
    tau_g(1:3,1) = Fb_g;
    

end

== matlab function guidance/Inverse Dynamics Controller/Inverse Dynamics/MATLAB Function ==
  data: eta input; Fb_g output; Fg input
function Fb_g = fcn(eta, Fg)
    R = quat2rotm(eta(4:7)');
    Fb_g = R' * Fg;
end

== matlab function guidance/Guidance/wpt ==
  data: idx input; xk_1 output; wpts input; xk output
function [xk_1, xk]= fcn(idx, wpts)
    [~, cs] = size(wpts);
    if idx < cs -1
        xk_1 = wpts(:,idx);
        xk = wpts(:,idx+1);
    else
        idx = cs -1;
        xk_1 = wpts(:,idx);
        xk = wpts(:,idx+1);
    end
end

== matlab function guidance/Guidance/SLERP Coeff ==
  data: slerp_coeff output; p_los input; etak input; etak_1 input; circle_of_acceptance_R input; interpolation_coeffs input
function slerp_coeff = fcn(p_los, etak, etak_1, circle_of_acceptance_R, interpolation_coeffs)
    d_eta = norm(etak(1:3) - etak_1(1:3));
    d_ratio = (norm(p_los - etak_1(1:3))+circle_of_acceptance_R)/d_eta;
    if d_ratio > 1
        d_ratio = 1;
    end
    slerp_coeff = polyval(interpolation_coeffs, d_ratio);
end

== matlab function guidance/Guidance/slerp ==
  data: q1 input; qd output size=4; q2 input; slerp_coeff input
function qd = fcn(q1, q2, slerp_coeff)
    q = slerp(quaternion(q1(4:7)'), quaternion(q2(4:7)'), slerp_coeff);
    [n, e1, e2, e3] = parts(q);
    qd = [n;e1;e2;e3];
end

== matlab function guidance/Guidance/MATLAB Function2 ==
  data: eta_d input; pdot_omd output; eta_d_1 input
function pdot_omd = fcn(eta_d, eta_d_1)
    pdot_d = eta_d(1:3) - eta_d_1(1:3);
    q_dot = eta_d(4:7) - eta_d_1(4:7);
    q = eta_d(4:7);
    q0 = q(1);
    q1 = q(2);
    q2 = q(3);
    q3 = q(4);
    E = [-q1 q0 -q3 q2;
         -q2 q3 q0 -q1;
         -q3 -q2 q1 q0];
    omd = 2*E*q_dot;
    pdot_omd = [pdot_d;omd];
end

== matlab function guidance/rot_params ==
  data: eta input size=7; eul_XYZ output
function eul_XYZ = fcn(eta)
    q = eta(4:7);
    eul_XYZ = quat2eul(q',"XYZ");
end

== matlab function guidance/Inverse Dynamics Controller/a controller/eta error ==
  data: eta input; delta_eta output size=6; etad input
function delta_eta = fcn(eta, etad)
    delta_pos = etad(1:3) - eta(1:3);
    q = quaternion(eta(4:7)');
    qd = quaternion(etad(4:7)');
    qe_de = conj(q)./(norm(q)^2) * qd;
    [~, e1, e2, e3] = parts(qe_de);
    epsilone_de = [e1;e2;e3];
    
    R = quat2rotm(q);
    delta_epsilon = R*epsilone_de;
    delta_eta = [delta_pos;delta_epsilon];

== matlab function guidance/Inverse Dynamics Controller/Body frame error velocities ==
  data: eta input; pdot_om input; pdot_om_b output size=6
function pdot_om_b = fcn(eta, pdot_om)
   R = quat2rotm(eta(4:7)');
   pdot_om_b = [R'*pdot_om(1:3); R'*pdot_om(4:6)];
end
